simulink model "Esm_ref"  (R2025b)
settings: Solver=FixedStepDiscrete  StartTime=0.0  StopTime=0.02  FixedStep=0.001  RelTol=1e-3
settings Model: Creator=leeyj  LastModifiedBy=leeyj

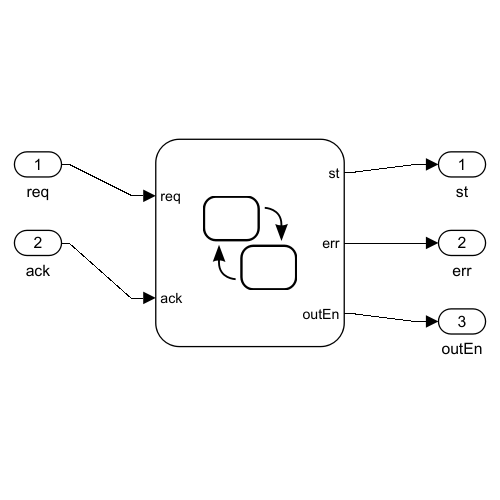
[thumbnail: Simulink's stored preview of the top-level diagram]
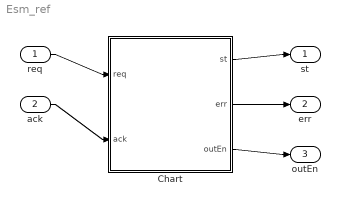
== system Esm_ref ==
  req : Inport  OutDataTypeStr=uint8
  ack : Inport  Port=2  OutDataTypeStr=boolean
  Chart : Stateflow chart  TreatAsAtomicUnit=on
  st : Outport
  err : Outport  Port=2
  outEn : Outport  Port=3
  wires:
  req/1 -> Chart/1(req)
  ack/1 -> Chart/2(ack)
  Chart/1(st) -> st/1
  Chart/2(err) -> err/1
  Chart/3(outEn) -> outEn/1

== stateflow chart Esm_ref/Chart ==
  settings: updateMethod=DISCRETE  sampleTime=0.001
  state Machine
    during: err = err && !ack;
    state Init
      entry: st = 1; outEn = 0;
      during: err = err || (req != 0 && req != 1 && req != 2);
    state PreOp
      entry: st = 2; outEn = 0;
      during: err = err || (req != 0 && req != 2 && req != 1 && req != 4);
    state SafeOp
      entry: st = 4; outEn = 0;
      during: err = err || (req != 0 && req != 4 && req != 1 && req != 2 && req != 8);
    state Op
      entry: st = 8; outEn = 1;
      during: err = err || (req != 0 && req != 8 && req != 1 && req != 2 && req != 4);
    Op -> Init [order 3] : [req == 1]
    SafeOp -> PreOp [order 2] : [req == 2 && !err]
    (default) -> Init
    SafeOp -> Op [order 1] : [req == 8 && !err]
    Init -> PreOp : [req == 2 && !err]
    Op -> PreOp [order 2] : [req == 2 && !err]
    Op -> SafeOp [order 1] : [req == 4 && !err]
    PreOp -> SafeOp [order 1] : [req == 4 && !err]
  SafeOp -> Init [order 3] : [req == 1]
  PreOp -> Init [order 2] : [req == 1]
  (default) -> Machine
  data: req input uint8; ack input boolean; st output uint8; err output boolean; outEn output boolean
